simulink model "Practica_asincronica"  (R2021a)
settings: Solver=ode23tb  StartTime=0.0  StopTime=10  MaxStep=500e-6  RelTol=1e-4  EnableMultiTasking=on
libraries: fl_lib x2, spsRMSLib x2, spsThreePhaseVIMeasurementLib x2, nesl_utility x2, spsThreePhaseProgrammableVoltageSourceLib x1, spsAsynchronousMachineSIUnitsLib x1, spsGroundLib x1, spsPowerLib x1, spsThreePhaseBreakerLib x1, spspowerguiLib x1
settings Model: ExtModeAutoUpdateStatusClock=off  Creator=MathWorks  LastModifiedBy=ontib
settings SolverCC: ZeroCrossAlgorithm=Adaptive  AlgebraicLoopSolver=TrustRegion
settings DataIOCC: LimitDataPoints=on  SaveFormat=Array  SignalLoggingSaveFormat=ModelDataLogs  ReturnWorkspaceOutputs=off
settings OptimizationCC: ExpressionDepthLimit=2147483647  InitFltsAndDblsToZero=on  EfficientMapNaN2IntZero=off  LifeSpan=inf
settings DebuggingCC: UnderspecifiedInitializationDetection=Classic  MergeDetectMultiDrivingBlocksExec=none  CheckExecutionContextPreStartOutputMsg=on  SignalResolutionControl=TryResolveAllWithWarning  SolverPrmCheckMsg=warning  MultiTaskDSMMsg=warning  MultiTaskCondExecSysMsg=none  SigSpecEnsureSampleTimeMsg=none  FcnCallInpInsideContextMsg=warning  StateNameClashWarn=warning  SFUnexpectedBacktrackingDiag=warning  SFNoUnconditionalDefaultTransitionDiag=warning  SFExecutionAtInitializationDiag=none  SFMachineParentedDataDiag=warning  ArithmeticOperatorsInVariantConditions=warning
settings HardwareCC: ProdBitPerPointer=32  ProdBitPerSizeT=32  ProdBitPerPtrDiffT=32  ProdLargestAtomicFloat=None  ProdIntDivRoundTo=Undefined  ProdEndianess=Unspecified  ProdWordSize=32  ProdHWDeviceType=32-bit Generic
settings ModelReferenceCC: PropagateSignalLabelsOutOfModel=off
settings SFSimCC: SimUseLocalCustomCode=off  CustomCodeUndefinedFunction=UseInterfaceOnly
settings RTWCC: RTWUseLocalCustomCode=off
settings CodeAppCC: StateflowObjectComments=on
settings GRTTargetCC: TargetFcnLib=ansi_tfl_tmw.mat  TargetLangStandard=C89/C90 (ANSI)  CombineOutputUpdateFcns=off  GRTInterface=on
settings ConfigComp: CovMetricSettings=dw  CovSaveCumulativeToWorkspaceVar=on  CovSaveSingleToWorkspaceVar=on  CovExternalEMLEnable=off  CovSFcnEnable=off
settings SimscapeCC: SimscapeNormalizeSystem=off

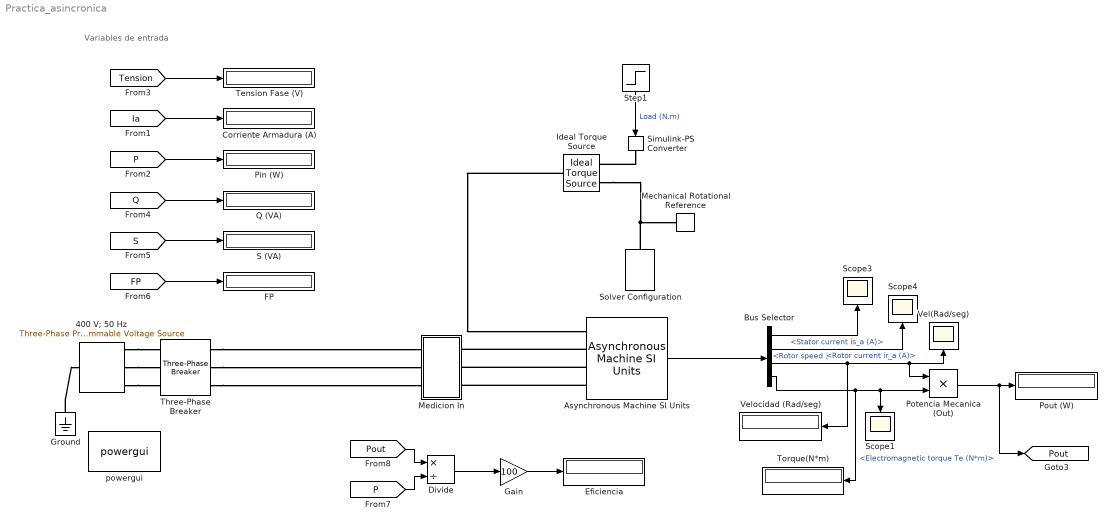
== system Practica_asincronica ==
  note: Variables de entrada
  400 V; 50 Hz : spsThreePhaseProgrammableVoltageSourceLib/Three-Phase Programmable Voltage Source  PositiveSequence="[400  0 50]"  VariationEntity=None  VariationType=Step  VariationTypeAlt=Step  VariationStep=0.5  VariationRate=10  VariationMagnitude=0.3  VariationFrequency=2  VariationTiming=[1 2]  VariationPhaseA=off  Amplitudes=[1 0.8 1.2 1.0]  TimeValues=[0 0.1 0.15 0.2]  HarmonicGeneration=off  HarmonicA=[3 0.2 -25 0]  HarmonicB=[2 0.15 35 2]  Timing="[0.05  3]"  BusType=swing  Pref=0  Qref=0  Qmin=-inf  Qmax=inf
  Asynchronous Machine SI Units : spsAsynchronousMachineSIUnitsLib/Asynchronous Machine SI Units  RotorType=Squirrel-cage  PresetModel=No  MechanicalLoad=Mechanical rotational port  ShowDetailedParameters=on  ReferenceFrame=Rotor  Units=SI  MeasurementBus=off  NominalParameters=[1.845e+04 400 50]  VoltageRatio=1  Stator=[0.5968 0.0003495]  Rotor=[0.6258 0.005473]  Cage1=[0.4155 0.002066]  Cage2=[0.4168 0.0003495]  Lm=0.0354  Mechanical=[0.05 0.005879 2]  PolePairs=2  InitialConditions=[0 0 0 0 0 0 0 0]  SimulateSaturation=off  Saturation=[14.03593122, 27.81365428, 53.79336849, 72.68890987, 97.98006896, 148.6815601, 215.7428561, 302.9841135, 428.7778367 ; 230, 322, 414, 460, 506, 552, 598, 644, 690]  LoadFlowParameters=1492000  TsPowergui=0  TsBlock=-1  IterativeModel=Trapezoidal non iterative  IterativeDiscreteModel=Trapezoidal non iterative  Pmec=1.492e+006
  Bus Selector : BusSelector  OutputSignals=Stator measurements.Stator current is_a (A),Rotor measurements.Rotor current ir_a (A),Mechanical.Rotor speed (wm),Mechanical.Electromagnetic torque Te (N*m)
  Corriente Armadura (A) : Display
      settings: Format=bank  Decimation=3
  Divide : Product  Inputs=*/
  Eficiencia : Display
  FP : Display
  Gain : Gain  Gain=100
  Ground : spsGroundLib/Ground  LConnTagsString=a
  Ideal Torque Source : fl_lib/Mechanical/Mechanical Sources/Ideal Torque Source
  Mechanical Rotational Reference : fl_lib/Mechanical/Rotational Elements/Mechanical Rotational Reference
  Medicion In : Subsystem
  Pin (W) : Display
      settings: Format=bank
  Potencia Mecanica (Out) : Product
  Pout (W) : Display
  Q (VA) : Display
      settings: Format=bank
  S (VA) : Display
      settings: Format=bank
  Scope1 : Scope
  Scope3 : Scope
  Scope4 : Scope
  Simulink-PS Converter : nesl_utility/Simulink-PS Converter  PhysicalDomain=network_engine_domain  SubClassName=ps_input  LeftPortType=input  RightPortType=output  PseudoPeriodic=off  Frequencies=[]  NoiseDistribution=none  NoiseParameters=[]  Unit=1  AffineConversion=off  FilteringAndDerivatives=provide  SimscapeFilterOrder=1  InputFilterTimeConstant=0.001  UdotUserProvided=0
      settings: SourceProductBaseCode=PW,SS
  Solver Configuration : nesl_utility/Solver Configuration  PhysicalDomain=network_engine_domain  SubClassName=solver  LeftPortType=input  RightPortType=generic  Tones=[]  Harmonics=[]  SimulateNoise=off  Profile=off  UseLocalSampling=off  EnableSwitchedLinearOptims=on  FrequencyDomain=off  UseCCode=off  RelTol=0.001  AbsTol=1e-06  MinStep=1e-09  ToWorkspace=off  RevertToSquareIcSolve=off  NumHomotopyIterations=100  PhasorMode=off  PhasorModeNumHarmonics=1  DoDC=off  ResidualTolerance=1e-09  UseLocalSolver=off  LocalSolverChoice=NE_BACKWARD_EULER_ADVANCER  LocalSolverSampleTime=0.001  DoFixedCost=off  MaxNonlinIter=3  MaxModeIter=2  ComputeImpulses=off  ImpulseIterations=2  LinearAlgebra=auto  EquationFormulation=NE_TIME_EF  DelaysMemoryBudget=1024  AutomaticFiltering=on  FilteringTimeConstant=0.001  PartitionStorageMethod=AS_NEEDED  PartitionMemoryBudget=1024  PartitionMethod=ROBUST
      settings: SourceProductBaseCode=PW,SS
  Step1 : Step  Time=6  After=-60  SampleTime=0
  Tension Fase (V) : Display
      settings: Format=bank  Decimation=3
  Three-Phase Breaker : spsThreePhaseBreakerLib/Three-Phase Breaker  InitialState=open  SwitchA=on  SwitchB=on  SwitchC=on  SwitchTimes=[0.01]  External=off  BreakerResistance=0.001  SnubberResistance=1e5  SnubberCapacitance=inf  Measurements=None
  Torque(N*m) : Display
  Vel(Rad/seg) : Scope
  Velocidad (Rad/seg) : Display
  powergui : spspowerguiLib/powergui  Priority=2  SimulationMode=Continuous  SampleTime=0  frequency=50  Iterations=50  frequencyindice=50  Pbase=100e6  ErrMax=1e-4  UnitsV=kV  UnitsW=MW  buscounter=0  FunctionMessages=off  echomessages=off  EnableUseOfTLC=off  CurrentSourceSwitches=off  DisableSnubberDevices=off  DisableRonSwitches=off  DisableVfSwitches=off  DisplayEquations=off  AutomaticDiscreteSolvers=off  SolverType=Tustin  Interpol=off  ExternalGateDelay=off  methode=off  Ts=0  x0status=blocks  SPID=on  SwTol=0  HookPort=off  NonlinearTolerance=1e-4  nMaxIteration=100  ContinueOnMaxIteration=off  RestoreLinks=warning  ResistiveCurrentMeasurement=off  Frange=[0:2:500]  Ylog=off  Xlog=on  ShowGrid=off  save=off  variable=ZData  structure=0  ZoomFFT=on  StartTime=0.0  cycles=1  DisplayStyle=1  fundamental=60  FreqAxis=off  MaxFrequency=1000  frequencyindicesteady=1  RmsSteady=1  display=off
  tag scope: Pout=global
  wires:
  Step1/1 -> Simulink-PS Converter/1  "Load (N.m)"
  [Tension] -> Tension Fase (V)/1
  [Ia] -> Corriente Armadura (A)/1
  [Q] -> Q (VA)/1
  [P] -> Pin (W)/1
  [S] -> S (VA)/1
  [FP] -> FP/1
  Asynchronous Machine SI Units/1 -> Bus Selector/1
  Potencia Mecanica (Out)/1 -> [Pout], Pout (W)/1
  Bus Selector/4 -> Torque(N*m)/1, Potencia Mecanica (Out)/2, Scope1/1  "<Electromagnetic torque Te (N*m)>"
  Bus Selector/3 -> Velocidad (Rad/seg)/1, Potencia Mecanica (Out)/1, Vel(Rad/seg)/1  "<Rotor speed (wm)>"
  Bus Selector/1 -> Scope3/1  "<Stator current is_a (A)>"
  Bus Selector/2 -> Scope4/1  "<Rotor current ir_a (A)>"
  Gain/1 -> Eficiencia/1
  Divide/1 -> Gain/1
  [P] -> Divide/2
  [Pout] -> Divide/1
  connections:
  400 V; 50 Hz/RConn1 -- Three-Phase Breaker/LConn1
  400 V; 50 Hz/RConn2 -- Three-Phase Breaker/LConn2
  400 V; 50 Hz/RConn3 -- Three-Phase Breaker/LConn3
  Ground/LConn1 -- 400 V; 50 Hz/LConn1
  Three-Phase Breaker/RConn1 -- Medicion In/LConn1
  Three-Phase Breaker/RConn2 -- Medicion In/LConn2
  Three-Phase Breaker/RConn3 -- Medicion In/LConn3
  Asynchronous Machine SI Units/LConn2 -- Medicion In/RConn1
  Asynchronous Machine SI Units/LConn3 -- Medicion In/RConn2
  Asynchronous Machine SI Units/LConn4 -- Medicion In/RConn3
  Solver Configuration/RConn1 -- Ideal Torque Source/RConn2 -- Mechanical Rotational Reference/LConn1
  Simulink-PS Converter/RConn1 -- Ideal Torque Source/RConn1
  Ideal Torque Source/LConn1 -- Asynchronous Machine SI Units/LConn1

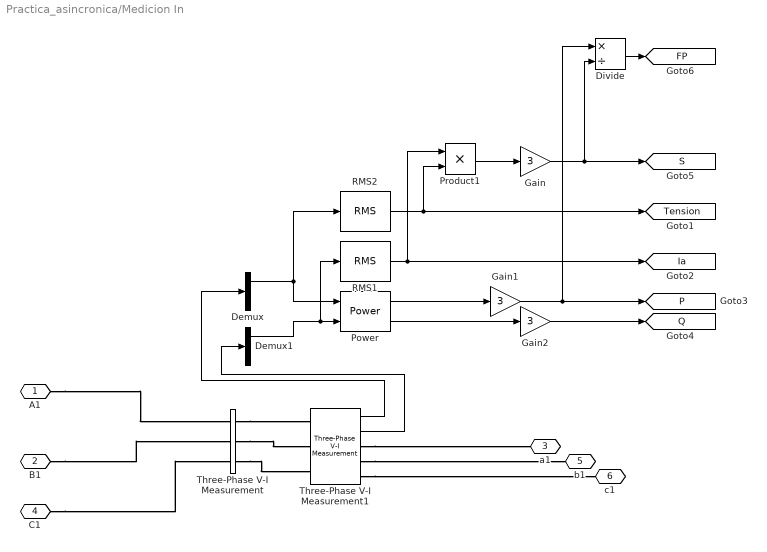
== system Practica_asincronica/Medicion In ==
  Demux : Demux  Outputs=3
  Demux1 : Demux  Outputs=3
  Divide : Product  Inputs=*/
  Gain : Gain  Gain=3
  Gain1 : Gain  Gain=3
  Gain2 : Gain  Gain=3
  Power : spsPowerLib/Power  Freq=50  Vinit=[1, 0]  Iinit=[1, 0]  Ts=0
      settings: SourceProductBaseCode=PS
  Product1 : Product
  RMS1 : spsRMSLib/RMS  TrueRMS=off  Freq=50  RMSInit=0  Ts=0
  RMS2 : spsRMSLib/RMS  TrueRMS=off  Freq=50  RMSInit=0  Ts=0
  Three-Phase V-I Measurement : spsThreePhaseVIMeasurementLib/Three-Phase V-I Measurement  VoltageMeasurement=phase-to-ground  SetLabelV=on  LabelV=Vabc  Vpu=off  VpuLL=off  CurrentMeasurement=no  SetLabelI=off  LabelI=Iabc  Ipu=off  Pbase=100e6  Vbase=500e3  OutputType=Complex  PhasorSimulation=off  PSBequivalent=0
  Three-Phase V-I Measurement1 : spsThreePhaseVIMeasurementLib/Three-Phase V-I Measurement  VoltageMeasurement=phase-to-ground  SetLabelV=off  LabelV=Vabc  Vpu=off  VpuLL=off  CurrentMeasurement=yes  SetLabelI=off  LabelI=Iabc  Ipu=off  Pbase=100e6  Vbase=500e3  OutputType=Complex  PhasorSimulation=off  PSBequivalent=0
  A1 : PMIOPort  Side=Left
  B1 : PMIOPort  Port=2  Side=Left
  a1 : PMIOPort  Port=3  Side=Right
  C1 : PMIOPort  Port=4  Side=Left
  b1 : PMIOPort  Port=5  Side=Right
  c1 : PMIOPort  Port=6  Side=Right
  tag scope: FP=global, Ia=global, P=global, Q=global, S=global, Tension=global
  wires:
  Gain2/1 -> [Q]
  Gain1/1 -> Divide/1, [P]
  RMS1/1 -> [Ia], Product1/1
  Power/2 -> Gain2/1
  Three-Phase V-I Measurement1/2 -> Demux1/1
  Three-Phase V-I Measurement1/1 -> Demux/1
  Demux/1 -> Power/1, RMS2/1
  RMS2/1 -> [Tension], Product1/2
  Product1/1 -> Gain/1
  Power/1 -> Gain1/1
  Demux1/1 -> RMS1/1, Power/2
  Gain/1 -> Divide/2, [S]
  Divide/1 -> [FP]
  connections:
  B1/RConn1 -- Three-Phase V-I Measurement/LConn2
  Three-Phase V-I Measurement/RConn2 -- Three-Phase V-I Measurement1/LConn2
  C1/RConn1 -- Three-Phase V-I Measurement/LConn3
  Three-Phase V-I Measurement1/RConn3 -- c1/RConn1
  Three-Phase V-I Measurement1/RConn2 -- b1/RConn1
  A1/RConn1 -- Three-Phase V-I Measurement/LConn1
  Three-Phase V-I Measurement/RConn1 -- Three-Phase V-I Measurement1/LConn1
  Three-Phase V-I Measurement/RConn3 -- Three-Phase V-I Measurement1/LConn3
  Three-Phase V-I Measurement1/RConn1 -- a1/RConn1
